simulink model "UGV_discr"  (R2016b)
settings: Solver=FixedStepAuto  StartTime=0.0  StopTime=20  FixedStep=ts_car  RelTol=1e-3
undefined symbols (not defined in the file or in its folder): DiscIntNeverNeededParam, ts_car, UGV_init, VehicleModel_discr
settings Model: Creator=nagym  LastModifiedBy=nagym
settings DataIOCC: ReturnWorkspaceOutputs=on
settings SFSimCC: SimUseLocalCustomCode=on
settings RTWCC: RTWUseLocalCustomCode=on

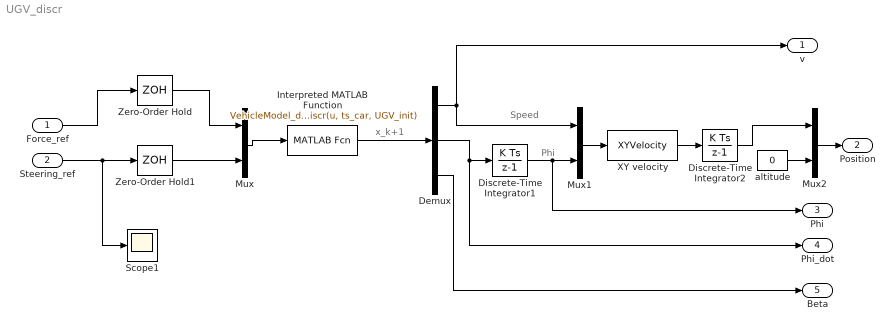
== system UGV_discr ==
  note: x_k+1
  note: Phi
  note: Speed
  Force_ref : Inport
  Steering_ref : Inport  Port=2
  Demux : Demux  Outputs=3
  Discrete-Time Integrator1 : DiscreteIntegrator  gainval=1  InitialConditionSetting=State (most efficient)  SampleTime=ts_car  ICPrevOutput=DiscIntNeverNeededParam  ICPrevScaledInput=DiscIntNeverNeededParam
  Discrete-Time Integrator2 : DiscreteIntegrator  gainval=1  InitialCondition=[0 0]  InitialConditionSetting=State (most efficient)  SampleTime=ts_car  ICPrevOutput=DiscIntNeverNeededParam  ICPrevScaledInput=DiscIntNeverNeededParam
  Interpreted MATLAB Function : MATLABFcn  MATLABFcn=VehicleModel_discr(u, ts_car, UGV_init)  OutputDimensions=3
  Mux : Mux  Inputs=2
  Mux1 : Mux  Inputs=2
  Mux2 : Mux  Inputs=2
  Scope1 : Scope
  XY velocity : MATLABFcn  MATLABFcn=XYVelocity  OutputDimensions=2
  Zero-Order Hold : ZeroOrderHold  SampleTime=ts_car
  Zero-Order Hold1 : ZeroOrderHold  SampleTime=ts_car
  altitude : Constant  Value=0
  v : Outport
  Position : Outport  Port=2
  Phi : Outport  Port=3
  Phi_dot : Outport  Port=4
  Beta : Outport  Port=5
  wires:
  Interpreted MATLAB Function/1 -> Demux/1
  Mux/1 -> Interpreted MATLAB Function/1
  Discrete-Time Integrator1/1 -> Phi/1, Mux1/2
  Demux/2 -> Discrete-Time Integrator1/1, Phi_dot/1
  XY velocity/1 -> Discrete-Time Integrator2/1
  Mux1/1 -> XY velocity/1
  Demux/3 -> Beta/1
  Discrete-Time Integrator2/1 -> Mux2/1
  Mux2/1 -> Position/1
  altitude/1 -> Mux2/2
  Demux/1 -> v/1, Mux1/1
  Force_ref/1 -> Zero-Order Hold/1
  Steering_ref/1 -> Scope1/1, Zero-Order Hold1/1
  Zero-Order Hold/1 -> Mux/1
  Zero-Order Hold1/1 -> Mux/2
